simulink model "enabledSubsystem"  (R2020b)
settings: Solver=VariableStepAuto  StartTime=0.0  StopTime=2  MaxStep=.001  RelTol=1e-3
settings Model: Creator=99003747  LastModifiedBy=99003747

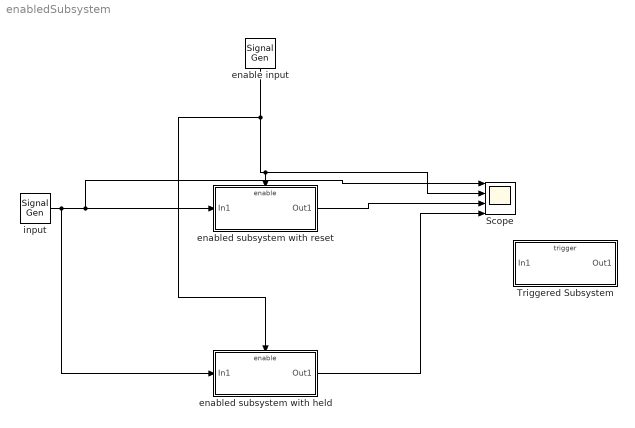
== system enabledSubsystem ==
  Scope : Scope  NumInputPorts=4
  Triggered Subsystem : Subsystem  TreatAsAtomicUnit=on
  "enable input " : SignalGenerator  WaveForm=square  Frequency=3
  enabled subsystem with held : Subsystem
  enabled subsystem with reset : Subsystem
  input : SignalGenerator
  wires:
  input/1 -> enabled subsystem with held/1(In1), Scope/1, enabled subsystem with reset/1(In1)
  "enable input "/1 -> enabled subsystem with held/Enable, Scope/2, enabled subsystem with reset/Enable
  enabled subsystem with reset/1(Out1) -> Scope/3
  enabled subsystem with held/1(Out1) -> Scope/4

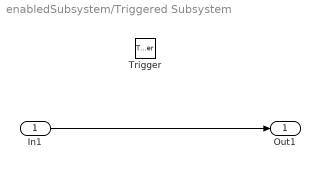
== system enabledSubsystem/Triggered Subsystem ==
  In1 : Inport
  Trigger : TriggerPort  VariantControl=Variant
  Out1 : Outport
  wires:
  In1/1 -> Out1/1

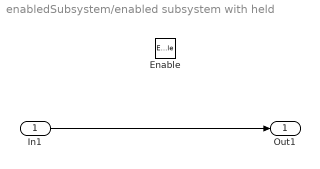
== system enabledSubsystem/enabled subsystem with held ==
  In1 : Inport
  Enable : EnablePort
  Out1 : Outport
  wires:
  In1/1 -> Out1/1

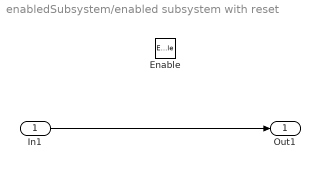
== system enabledSubsystem/enabled subsystem with reset ==
  In1 : Inport
  Enable : EnablePort  StatesWhenEnabling=reset
  Out1 : Outport
  wires:
  In1/1 -> Out1/1
